simulink model "egnition_New_updated_shiva"  (R2019b)
settings: Solver=ode1  StartTime=0.0  StopTime=170  FixedStep=0.01  RelTol=1e-3
undefined symbols (not defined in the file or in its folder): BezierCurves, BezierLength, Constants, Driver, Ln, magnitude, v31
libraries: simulink_extras x3, simulink x2
(part 2 of 2)

== system egnition_New_updated_shiva/Tire Forces /Tire Model/co efficient of friction calculation ==
  "Resultant Slip " : Inport
  Fz : Inport  Port=2
  Bus Creator : BusCreator  Inputs=4
  Bus Creator1 : BusCreator  Inputs=4
  Bus Creator2 : BusCreator  Inputs=2
  Bus Selector : BusSelector  OutputSignals=Slip:L_FL,Slip:L_FR,Slip:L_RL,Slip:L_RR,Slip:S_FL,Slip:S_FR,Slip:S_RL,Slip:S_RR
  Bus Selector1 : BusSelector  OutputSignals=Resultant Slip FL,Resultant Slip FR,Resultant Slip RL,Resultant Slip RR
  Bus Selector2 : BusSelector  OutputSignals=Longitudinal_and_side_Slip,Resultant_Slip
  Bus Selector3 : BusSelector  OutputSignals=Fz_Dynamic.FZD_FL,Fz_Dynamic.FZD_FR,Fz_Dynamic.FZD_RL,Fz_Dynamic.FZD_RR
  Constant : Constant  Value=Constants.other_param.Friction_Tuning_Parameter
  Demux : Demux  Outputs=8
  MATLAB Code : MATLAB Function  TreatAsAtomicUnit=on
  Mew : Outport  VectorParamsAs1DForOutWhenUnconnected=off
  wires:
  Bus Selector2/1 -> Bus Selector/1  "<Longitudinal_and_side_Slip>"
  Bus Selector2/2 -> Bus Selector1/1  "<Resultant_Slip>"
  Bus Selector3/4 -> MATLAB Code/16(FZD_RR)  "<FZD_RR>"
  Bus Selector3/3 -> MATLAB Code/15(FZD_RL)  "<FZD_RL>"
  Bus Selector3/2 -> MATLAB Code/14(FZD_FR)  "<FZD_FR>"
  Bus Selector3/1 -> MATLAB Code/13(FZD_FL)  "<FZD_FL>"
  MATLAB Code/1(y) -> Demux/1
  Bus Selector1/1 -> MATLAB Code/9(SlipR_FL)  "<Resultant Slip FL>"
  Bus Selector1/2 -> MATLAB Code/10(SlipR_FR)  "<Resultant Slip FR>"
  Bus Selector1/3 -> MATLAB Code/11(SlipR_RL)  "<Resultant Slip RL>"
  Bus Selector1/4 -> MATLAB Code/12(SlipR_RR)  "<Resultant Slip RR>"
  Bus Selector/8 -> MATLAB Code/8(SlipS_RR)  "<Slip:S_RR>"
  Bus Selector/7 -> MATLAB Code/7(SlipS_RL)  "<Slip:S_RL>"
  Bus Selector/6 -> MATLAB Code/6(SlipS_FR)  "<Slip:S_FR>"
  Bus Selector/5 -> MATLAB Code/5(SlipS_FL)  "<Slip:S_FL>"
  Bus Selector/4 -> MATLAB Code/4(SlipL_RR)  "<Slip:L_RR>"
  Bus Selector/3 -> MATLAB Code/3(SlipL_RL)  "<Slip:L_RL>"
  Bus Selector/2 -> MATLAB Code/2(SlipL_FR)  "<Slip:L_FR>"
  Bus Selector/1 -> MATLAB Code/1(SlipL_FL)  "<Slip:L_FL>"
  Bus Creator/1 -> Bus Creator2/1  "Mew(l)"
  Bus Creator1/1 -> Bus Creator2/2  "Mew(s)"
  Bus Creator2/1 -> Mew/1
  "Resultant Slip "/1 -> Bus Selector2/1
  Demux/1 -> Bus Creator/1  "Mew(l)_FL"
  Demux/2 -> Bus Creator/2  "Mew(l)_FR"
  Demux/3 -> Bus Creator/3  "Mew(l)_RL"
  Demux/4 -> Bus Creator/4  "Mew(l)_RR"
  Demux/5 -> Bus Creator1/1  "Mew(s)_FL"
  Demux/6 -> Bus Creator1/2  "Mew(s)_FR"
  Demux/7 -> Bus Creator1/3  "Mew(s)_RL"
  Demux/8 -> Bus Creator1/4  "Mew(s)_RR"
  Constant/1 -> MATLAB Code/17(Friction_Tuning_parameter)
  Fz/1 -> Bus Selector3/1

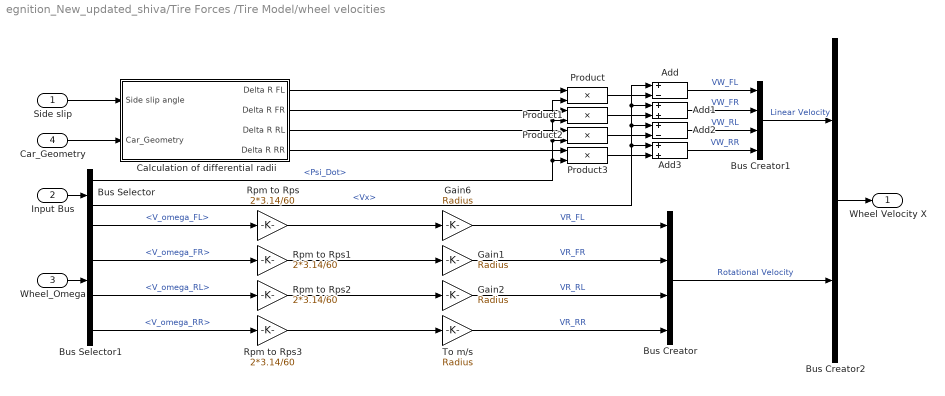
== system egnition_New_updated_shiva/Tire Forces /Tire Model/wheel velocities  ==
  "Side slip " : Inport
  Input Bus : Inport  Port=2
  Wheel_Omega : Inport  Port=3
  Car_Geometry : Inport  Port=4
  Add : Sum  Inputs=+-
  Add1 : Sum
  Add2 : Sum  Inputs=+-
  Add3 : Sum
  Bus Creator : BusCreator  Inputs=4
  Bus Creator1 : BusCreator  Inputs=4
  Bus Creator2 : BusCreator  Inputs=2
  Bus Selector : BusSelector  OutputSignals=Velocity.Psi_Dot,Velocity.Vx
  Bus Selector1 : BusSelector  OutputSignals=V_omega_FL,V_omega_FR,V_omega_RL,V_omega_RR
  Calculation of differential radii : Subsystem
  Gain1 : Gain  Gain=Radius
  Gain2 : Gain  Gain=Radius
  Gain6 : Gain  Gain=Radius
  Product{,1..3} (4 alike) : Product
  Rpm to Rps{,1..3} (4 alike) : Gain  Gain=2*3.14/60
  To m/s : Gain  Gain=Radius
  Wheel Velocity X : Outport  VectorParamsAs1DForOutWhenUnconnected=off
  wires:
  Car_Geometry/1 -> Calculation of differential radii/2(Car_Geometry)
  Wheel_Omega/1 -> Bus Selector1/1
  To m/s/1 -> Bus Creator/4  "VR_RR"
  Gain2/1 -> Bus Creator/3  "VR_RL"
  Gain1/1 -> Bus Creator/2  "VR_FR"
  Gain6/1 -> Bus Creator/1  "VR_FL"
  Input Bus/1 -> Bus Selector/1
  Add3/1 -> Bus Creator1/4  "VW_RR"
  Add2/1 -> Bus Creator1/3  "VW_RL"
  Add1/1 -> Bus Creator1/2  "VW_FR"
  Add/1 -> Bus Creator1/1  "VW_FL"
  Bus Selector/2 -> Add3/1, Add2/1, Add1/1, Add/1  "<Vx>"
  Product3/1 -> Add3/2
  Product2/1 -> Add2/2
  Product1/1 -> Add1/2
  Product/1 -> Add/2
  Bus Selector/1 -> Product3/2, Product2/2, Product1/2, Product/2  "<Psi_Dot>"
  Calculation of differential radii/4(Delta R RR) -> Product3/1
  Calculation of differential radii/3(Delta R RL) -> Product2/1
  Calculation of differential radii/2(Delta R FR) -> Product1/1
  Calculation of differential radii/1(Delta R FL) -> Product/1
  "Side slip "/1 -> Calculation of differential radii/1(Side slip angle)
  Bus Creator1/1 -> Bus Creator2/1  "Linear Velocity"
  Bus Creator/1 -> Bus Creator2/2  "Rotational Velocity"
  Bus Creator2/1 -> Wheel Velocity X/1
  Bus Selector1/1 -> Rpm to Rps/1  "<V_omega_FL>"
  Bus Selector1/2 -> Rpm to Rps1/1  "<V_omega_FR>"
  Bus Selector1/3 -> Rpm to Rps2/1  "<V_omega_RL>"
  Bus Selector1/4 -> Rpm to Rps3/1  "<V_omega_RR>"
  Rpm to Rps/1 -> Gain6/1
  Rpm to Rps1/1 -> Gain1/1
  Rpm to Rps2/1 -> Gain2/1
  Rpm to Rps3/1 -> To m/s/1

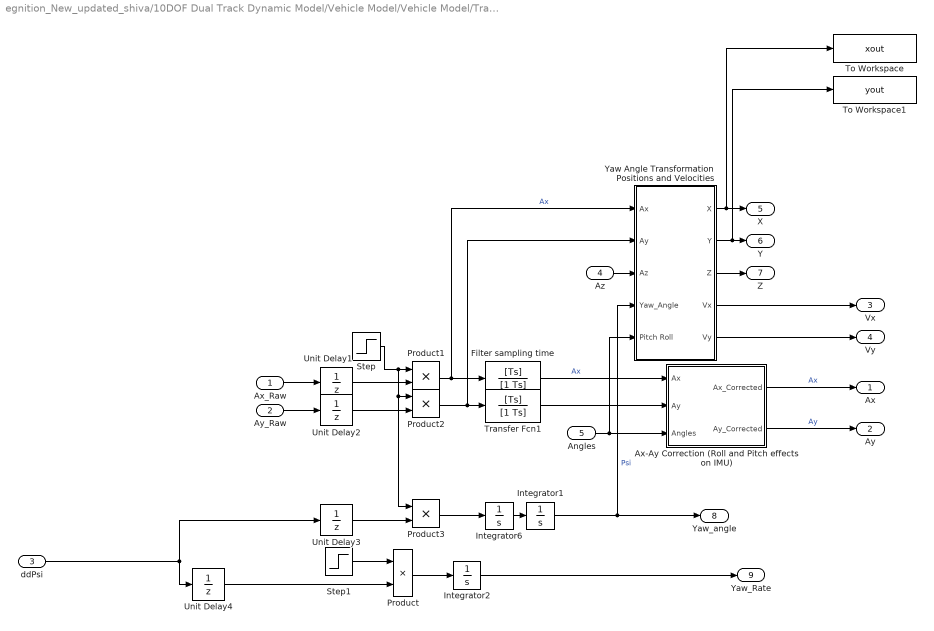
== system egnition_New_updated_shiva/10DOF Dual Track Dynamic Model/Vehicle Model/Vehicle Model/Transformation from Raw States to Car States ==
  Ax_Raw : Inport
  Ay_Raw : Inport  Port=2
  ddPsi : Inport  Port=3
  Az : Inport  Port=4
  Angles : Inport  Port=5
  Ax-Ay Correction (Roll and Pitch effects on IMU) : Subsystem
  Filter sampling time : TransferFcn  Numerator=[Ts]  Denominator=[1 Ts]
  Integrator1 : Integrator
  Integrator2 : Integrator  InitialCondition=0.0000000001
  Integrator6 : Integrator
  Product{,1..3} (4 alike) : Product
  Step : Step  Time=2
  Step1 : Step  Time=2.00000
  To Workspace : ToWorkspace  VariableName=xout  SampleTime=-1
  To Workspace1 : ToWorkspace  VariableName=yout  SampleTime=-1
  Transfer Fcn1 : TransferFcn  Numerator=[Ts]  Denominator=[1 Ts]
  Unit Delay1 : UnitDelay  SampleTime=-1  HasFrameUpgradeWarning=on
  Unit Delay2 : UnitDelay  SampleTime=-1  HasFrameUpgradeWarning=on
  Unit Delay3 : UnitDelay  SampleTime=-1  HasFrameUpgradeWarning=on
  Unit Delay4 : UnitDelay  InitialCondition=0.1  SampleTime=-1  HasFrameUpgradeWarning=on
  "Yaw Angle Transformation Positions and Velocities " : Subsystem
  Ax : Outport  VectorParamsAs1DForOutWhenUnconnected=off
  Ay : Outport  Port=2  VectorParamsAs1DForOutWhenUnconnected=off
  Vx : Outport  Port=3  VectorParamsAs1DForOutWhenUnconnected=off
  Vy : Outport  Port=4  VectorParamsAs1DForOutWhenUnconnected=off
  X : Outport  Port=5  VectorParamsAs1DForOutWhenUnconnected=off
  Y : Outport  Port=6  VectorParamsAs1DForOutWhenUnconnected=off
  Z : Outport  Port=7  VectorParamsAs1DForOutWhenUnconnected=off
  Yaw_angle : Outport  Port=8  VectorParamsAs1DForOutWhenUnconnected=off
  Yaw_Rate : Outport  Port=9  VectorParamsAs1DForOutWhenUnconnected=off
  wires:
  Ax-Ay Correction (Roll and Pitch effects on IMU)/2("Ay_Corrected ") -> Ay/1  "Ay"
  Ax-Ay Correction (Roll and Pitch effects on IMU)/1(Ax_Corrected) -> Ax/1  "Ax"
  Integrator2/1 -> Yaw_Rate/1
  Product/1 -> Integrator2/1
  Unit Delay4/1 -> Product/2
  ddPsi/1 -> Unit Delay3/1, Unit Delay4/1
  "Yaw Angle Transformation Positions and Velocities "/3(Z) -> Z/1
  Az/1 -> "Yaw Angle Transformation Positions and Velocities "/3("Az ")
  Unit Delay1/1 -> Product1/2
  Unit Delay2/1 -> Product2/2
  Unit Delay3/1 -> Product3/2
  Step/1 -> Product1/1, Product2/1, Product3/1
  Product3/1 -> Integrator6/1
  Ax_Raw/1 -> Unit Delay1/1
  Ay_Raw/1 -> Unit Delay2/1
  Integrator6/1 -> Integrator1/1
  "Yaw Angle Transformation Positions and Velocities "/2(Y) -> To Workspace1/1, Y/1
  "Yaw Angle Transformation Positions and Velocities "/1(X) -> To Workspace/1, X/1
  Integrator1/1 -> "Yaw Angle Transformation Positions and Velocities "/4(Yaw_Angle), Yaw_angle/1  "Psi"
  Step1/1 -> Product/1
  Product1/1 -> Filter sampling time/1, "Yaw Angle Transformation Positions and Velocities "/1(Ax)  "Ax"
  Angles/1 -> Ax-Ay Correction (Roll and Pitch effects on IMU)/3("Angles "), "Yaw Angle Transformation Positions and Velocities "/5("Pitch Roll ")
  Product2/1 -> Transfer Fcn1/1, "Yaw Angle Transformation Positions and Velocities "/2(Ay)
  Filter sampling time/1 -> Ax-Ay Correction (Roll and Pitch effects on IMU)/1(Ax)  "Ax"
  Transfer Fcn1/1 -> Ax-Ay Correction (Roll and Pitch effects on IMU)/2(Ay)
  "Yaw Angle Transformation Positions and Velocities "/4(Vx) -> Vx/1
  "Yaw Angle Transformation Positions and Velocities "/5(Vy) -> Vy/1

== system egnition_New_updated_shiva/Driver Model/lateral Controller/Subsystem/dynamic Stanely ==
  ey : Inport
  v : Inport  Port=2
  r_meas : Inport  Port=3
  r_trj : Inport  Port=4
  Yaw_c : Inport  Port=5
  Corrective_dynamic_Terms : Subsystem
  IC : InitialCondition  Value=0
  Kinematic_controller : Subsystem
  Radians to Degrees1 : simulink_extras/Transformations/Radians to Degrees
  Sum1 : Sum  Inputs=|++
  dynamic_steer : Outport
  wires:
  r_meas/1 -> Corrective_dynamic_Terms/1(r_meas)
  r_trj/1 -> Corrective_dynamic_Terms/5(r_trj)
  Corrective_dynamic_Terms/1(steer_correction) -> Sum1/2
  Sum1/1 -> Radians to Degrees1/1, Corrective_dynamic_Terms/2(steer)
  ey/1 -> Kinematic_controller/1(ey)
  v/1 -> Kinematic_controller/2(v), Corrective_dynamic_Terms/4(v)
  Kinematic_controller/1(delta_fb) -> Sum1/1
  Yaw_c/1 -> Corrective_dynamic_Terms/3(yaw_c)
  Radians to Degrees1/1 -> IC/1
  IC/1 -> dynamic_steer/1

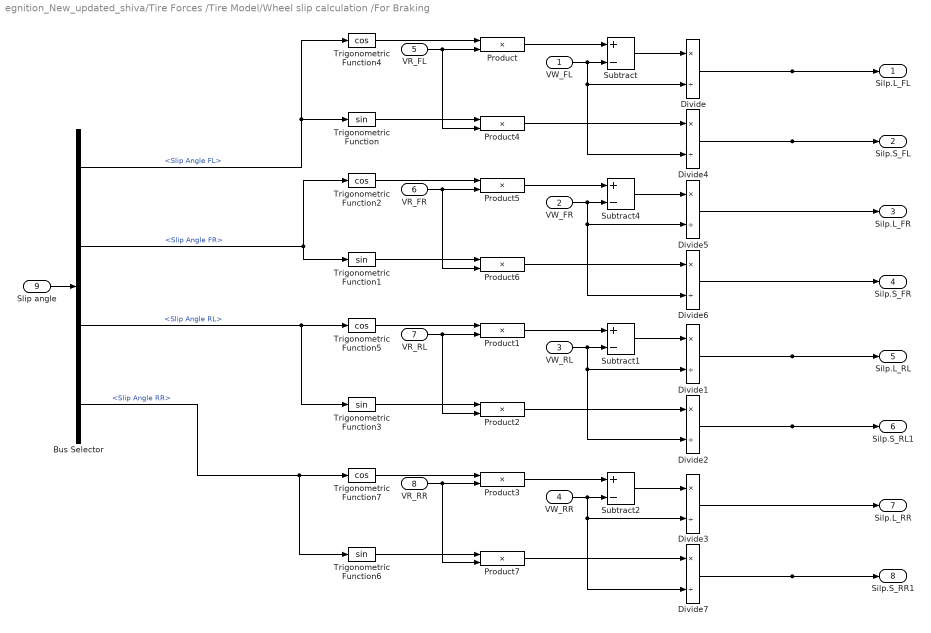
== system egnition_New_updated_shiva/Tire Forces /Tire Model/Wheel slip calculation /For Braking ==
  "VW_FL " : Inport
  VW_FR : Inport  Port=2
  VW_RL : Inport  Port=3
  VW_RR : Inport  Port=4
  VR_FL : Inport  Port=5
  VR_FR : Inport  Port=6
  VR_RL : Inport  Port=7
  "VR_RR " : Inport  Port=8
  "Slip angle " : Inport  Port=9
  Bus Selector : BusSelector  OutputSignals=Slip Angle FL,Slip Angle FR,Slip Angle RL,Slip Angle RR
  Divide{,1..7} (8 alike) : Product  Inputs=*/
  Product{,1..7} (8 alike) : Product
  Subtract{,1..2,4} (4 alike) : Sum  Inputs=+-
  Trigonometric Function{,1,3,6} (4 alike) : Trigonometry
  Trigonometric Function{2,4..5,7} (4 alike) : Trigonometry  Operator=cos
  Silp.L_FL : Outport  VectorParamsAs1DForOutWhenUnconnected=off
  Silp.S_FL : Outport  Port=2  VectorParamsAs1DForOutWhenUnconnected=off
  Silp.L_FR : Outport  Port=3  VectorParamsAs1DForOutWhenUnconnected=off
  Silp.S_FR : Outport  Port=4  VectorParamsAs1DForOutWhenUnconnected=off
  Silp.L_RL : Outport  Port=5  VectorParamsAs1DForOutWhenUnconnected=off
  Silp.S_RL1 : Outport  Port=6  VectorParamsAs1DForOutWhenUnconnected=off
  Silp.L_RR : Outport  Port=7  VectorParamsAs1DForOutWhenUnconnected=off
  Silp.S_RR1 : Outport  Port=8  VectorParamsAs1DForOutWhenUnconnected=off
  wires:
  "Slip angle "/1 -> Bus Selector/1
  Bus Selector/4 -> Trigonometric Function6/1, Trigonometric Function7/1  "<Slip Angle RR>"
  VW_RR/1 -> Subtract2/2, Divide3/2, Divide7/2
  Product7/1 -> Divide7/1
  "VR_RR "/1 -> Product3/2, Product7/2
  Product3/1 -> Subtract2/1
  Trigonometric Function6/1 -> Product7/1
  Subtract2/1 -> Divide3/1
  Trigonometric Function7/1 -> Product3/1
  VW_RL/1 -> Subtract1/2, Divide1/2, Divide2/2
  Product2/1 -> Divide2/1
  VR_RL/1 -> Product1/2, Product2/2
  Product1/1 -> Subtract1/1
  Trigonometric Function3/1 -> Product2/1
  Subtract1/1 -> Divide1/1
  Bus Selector/3 -> Trigonometric Function5/1, Trigonometric Function3/1  "<Slip Angle RL>"
  Trigonometric Function5/1 -> Product1/1
  Product5/1 -> Subtract4/1
  VW_FR/1 -> Subtract4/2, Divide5/2, Divide6/2
  Bus Selector/2 -> Trigonometric Function1/1, Trigonometric Function2/1  "<Slip Angle FR>"
  Trigonometric Function2/1 -> Product5/1
  VR_FR/1 -> Product5/2, Product6/2
  Subtract4/1 -> Divide5/1
  Trigonometric Function1/1 -> Product6/1
  Product6/1 -> Divide6/1
  Product4/1 -> Divide4/1
  Trigonometric Function/1 -> Product4/1
  "VW_FL "/1 -> Subtract/2, Divide/2, Divide4/2
  Product/1 -> Subtract/1
  Subtract/1 -> Divide/1
  VR_FL/1 -> Product/2, Product4/2
  Bus Selector/1 -> Trigonometric Function/1, Trigonometric Function4/1  "<Slip Angle FL>"
  Trigonometric Function4/1 -> Product/1
  Divide/1 -> Silp.L_FL/1
  Divide4/1 -> Silp.S_FL/1
  Divide5/1 -> Silp.L_FR/1
  Divide6/1 -> Silp.S_FR/1
  Divide1/1 -> Silp.L_RL/1
  Divide2/1 -> Silp.S_RL1/1
  Divide3/1 -> Silp.L_RR/1
  Divide7/1 -> Silp.S_RR1/1

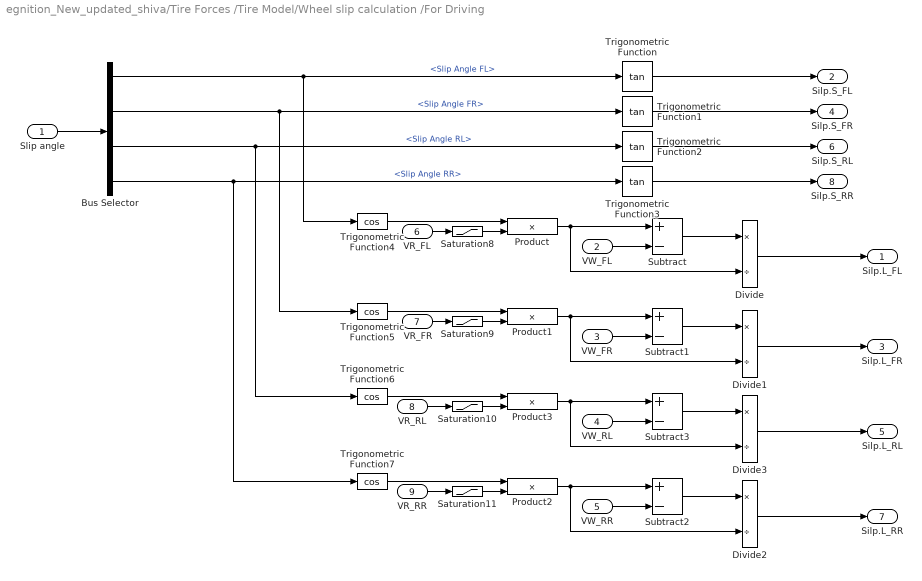
== system egnition_New_updated_shiva/Tire Forces /Tire Model/Wheel slip calculation /For Driving ==
  "Slip angle " : Inport
  "VW_FL " : Inport  Port=2
  VW_FR : Inport  Port=3
  VW_RL : Inport  Port=4
  VW_RR : Inport  Port=5
  VR_FL : Inport  Port=6
  VR_FR : Inport  Port=7
  VR_RL : Inport  Port=8
  "VR_RR " : Inport  Port=9
  Bus Selector : BusSelector  OutputSignals=Slip Angle FL,Slip Angle FR,Slip Angle RL,Slip Angle RR
  Divide{,1..3} (4 alike) : Product  Inputs=*/
  Product{,1..3} (4 alike) : Product
  Saturation{8..11} (4 alike) : Saturate  UpperLimit=500  LowerLimit=0.1
  Subtract{,1..3} (4 alike) : Sum  Inputs=+-
  Trigonometric Function{,1..3} (4 alike) : Trigonometry  Operator=tan
  Trigonometric Function{4..7} (4 alike) : Trigonometry  Operator=cos
  Silp.L_FL : Outport  VectorParamsAs1DForOutWhenUnconnected=off
  Silp.S_FL : Outport  Port=2  VectorParamsAs1DForOutWhenUnconnected=off
  Silp.L_FR : Outport  Port=3  VectorParamsAs1DForOutWhenUnconnected=off
  Silp.S_FR : Outport  Port=4  VectorParamsAs1DForOutWhenUnconnected=off
  Silp.L_RL : Outport  Port=5  VectorParamsAs1DForOutWhenUnconnected=off
  Silp.S_RL : Outport  Port=6  VectorParamsAs1DForOutWhenUnconnected=off
  Silp.L_RR : Outport  Port=7  VectorParamsAs1DForOutWhenUnconnected=off
  Silp.S_RR : Outport  Port=8  VectorParamsAs1DForOutWhenUnconnected=off
  wires:
  Saturation11/1 -> Product2/2
  Saturation10/1 -> Product3/2
  Saturation9/1 -> Product1/2
  Saturation8/1 -> Product/2
  Divide2/1 -> Silp.L_RR/1
  Divide3/1 -> Silp.L_RL/1
  Divide1/1 -> Silp.L_FR/1
  Divide/1 -> Silp.L_FL/1
  Trigonometric Function3/1 -> Silp.S_RR/1
  Trigonometric Function2/1 -> Silp.S_RL/1
  Trigonometric Function1/1 -> Silp.S_FR/1
  Trigonometric Function/1 -> Silp.S_FL/1
  "Slip angle "/1 -> Bus Selector/1
  Trigonometric Function5/1 -> Product1/1
  Product3/1 -> Subtract3/1, Divide3/2
  Trigonometric Function7/1 -> Product2/1
  VW_RR/1 -> Subtract2/2
  Product2/1 -> Subtract2/1, Divide2/2
  "VR_RR "/1 -> Saturation11/1
  Product1/1 -> Subtract1/1, Divide1/2
  Trigonometric Function6/1 -> Product3/1
  VR_RL/1 -> Saturation10/1
  Subtract1/1 -> Divide1/1
  Subtract2/1 -> Divide2/1
  VR_FR/1 -> Saturation9/1
  VW_RL/1 -> Subtract3/2
  VW_FR/1 -> Subtract1/2
  Subtract3/1 -> Divide3/1
  "VW_FL "/1 -> Subtract/2
  Product/1 -> Subtract/1, Divide/2
  Subtract/1 -> Divide/1
  VR_FL/1 -> Saturation8/1
  Bus Selector/4 -> Trigonometric Function3/1, Trigonometric Function7/1  "<Slip Angle RR>"
  Bus Selector/3 -> Trigonometric Function2/1, Trigonometric Function6/1  "<Slip Angle RL>"
  Bus Selector/2 -> Trigonometric Function1/1, Trigonometric Function5/1  "<Slip Angle FR>"
  Bus Selector/1 -> Trigonometric Function/1, Trigonometric Function4/1  "<Slip Angle FL>"
  Trigonometric Function4/1 -> Product/1

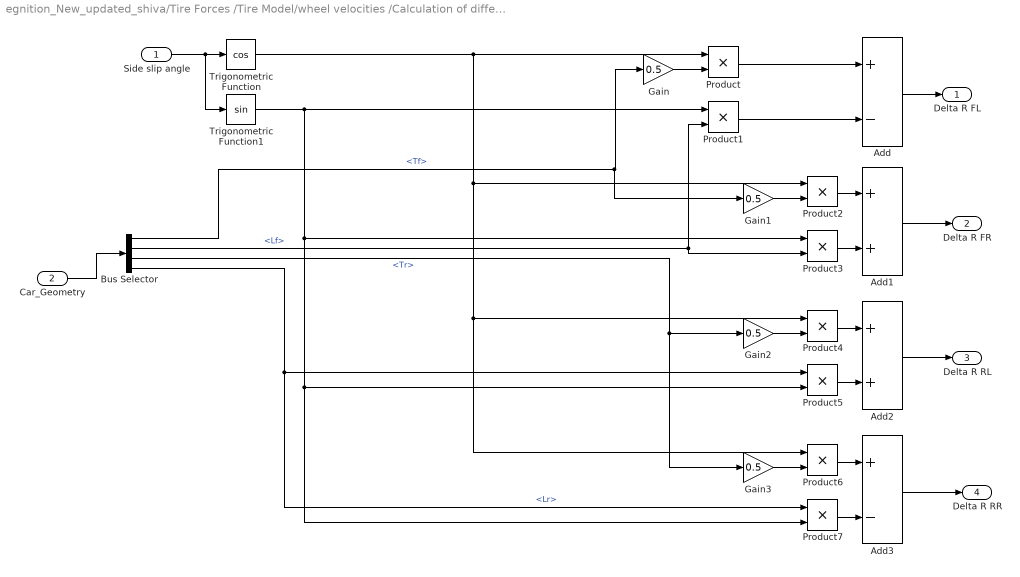
== system egnition_New_updated_shiva/Tire Forces /Tire Model/wheel velocities /Calculation of differential radii ==
  Side slip angle : Inport
  Car_Geometry : Inport  Port=2
  Add : Sum  Inputs=+-
  Add1 : Sum
  Add2 : Sum
  Add3 : Sum  Inputs=+-
  Bus Selector : BusSelector  OutputSignals=Tf,Lf,Tr,Lr
  Gain{,1..3} (4 alike) : Gain  Gain=0.5
  Product{,1..7} (8 alike) : Product
  Trigonometric Function : Trigonometry  Operator=cos
  Trigonometric Function1 : Trigonometry
  Delta R FL : Outport  VectorParamsAs1DForOutWhenUnconnected=off
  Delta R FR : Outport  Port=2  VectorParamsAs1DForOutWhenUnconnected=off
  Delta R RL : Outport  Port=3  VectorParamsAs1DForOutWhenUnconnected=off
  Delta R RR : Outport  Port=4  VectorParamsAs1DForOutWhenUnconnected=off
  wires:
  Car_Geometry/1 -> Bus Selector/1
  Add3/1 -> Delta R RR/1
  Add2/1 -> Delta R RL/1
  Add1/1 -> Delta R FR/1
  Add/1 -> Delta R FL/1
  Bus Selector/4 -> Product5/1, Product7/1  "<Lr>"
  Bus Selector/3 -> Gain2/1, Gain3/1  "<Tr>"
  Gain3/1 -> Product6/2
  Product6/1 -> Add3/1
  Product7/1 -> Add3/2
  Gain2/1 -> Product4/2
  Product4/1 -> Add2/1
  Product5/1 -> Add2/2
  Gain1/1 -> Product2/2
  Product2/1 -> Add1/1
  Product3/1 -> Add1/2
  Product/1 -> Add/1
  Product1/1 -> Add/2
  Trigonometric Function1/1 -> Product1/1, Product3/1, Product7/2, Product5/2
  Bus Selector/2 -> Product1/2, Product3/2  "<Lf>"
  Trigonometric Function/1 -> Product/1, Product2/1, Product6/1, Product4/1
  Gain/1 -> Product/2
  Bus Selector/1 -> Gain/1, Gain1/1  "<Tf>"
  Side slip angle/1 -> Trigonometric Function/1, Trigonometric Function1/1

== system egnition_New_updated_shiva/10DOF Dual Track Dynamic Model/Vehicle Model/Vehicle Model/Transformation from Raw States to Car States/Ax-Ay Correction (Roll and Pitch effects on IMU) ==
  Ax : Inport
  Ay : Inport  Port=2
  "Angles " : Inport  Port=3
  Add : Sum
  Add1 : Sum  Inputs=+-
  Bus Selector : BusSelector  OutputSignals=Theta,Phi
  Cos : Trigonometry  Operator=cos
  Gain : Gain  Gain=9.81
  Gain1 : Gain  Gain=9.81
  Product : Product
  Sin : Trigonometry
  Sin1 : Trigonometry
  Ax_Corrected : Outport  VectorParamsAs1DForOutWhenUnconnected=off
  "Ay_Corrected " : Outport  Port=2  VectorParamsAs1DForOutWhenUnconnected=off
  wires:
  "Angles "/1 -> Bus Selector/1
  Bus Selector/1 -> Sin/1, Cos/1  "<Theta>"
  Bus Selector/2 -> Sin1/1  "<Phi>"
  Ax/1 -> Add/1
  Sin/1 -> Gain/1
  Gain/1 -> Add/2
  Cos/1 -> Product/1
  Sin1/1 -> Product/2
  Gain1/1 -> Add1/2
  Ay/1 -> Add1/1
  Add/1 -> Ax_Corrected/1
  Add1/1 -> "Ay_Corrected "/1
  Product/1 -> Gain1/1

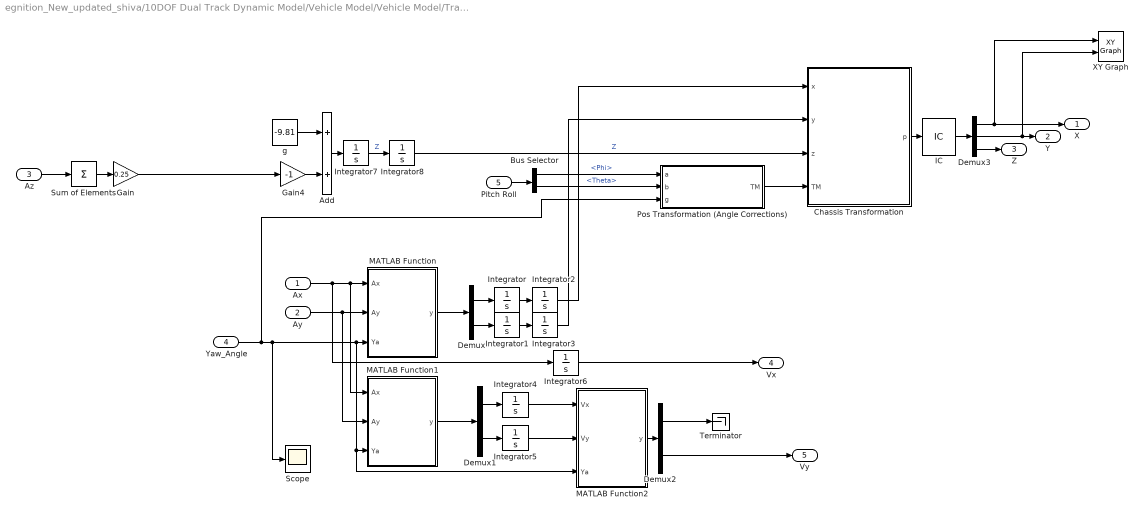
== system egnition_New_updated_shiva/10DOF Dual Track Dynamic Model/Vehicle Model/Vehicle Model/Transformation from Raw States to Car States/Yaw Angle Transformation Positions and Velocities  ==
  Ax : Inport
  Ay : Inport  Port=2
  "Az " : Inport  Port=3
  Yaw_Angle : Inport  Port=4
  "Pitch Roll " : Inport  Port=5
  Add : Sum
  Bus Selector : BusSelector  OutputSignals=Phi,Theta
  Chassis Transformation : MATLAB Function  TreatAsAtomicUnit=on
  Demux : Demux  Outputs=2
  Demux1 : Demux  Outputs=2
  Demux2 : Demux  Outputs=2
  Demux3 : Demux  Outputs=3
  Gain : Gain  Gain=0.25
  Gain4 : Gain  Gain=-1
  IC : InitialCondition  Value=[Constants.initial_param.X0;Constants.initial_param.Y0;Constants.initial_param.Z0]
  Integrator{,1,4..5,7} (5 alike) : Integrator
  Integrator2 : Integrator  InitialCondition=Constants.initial_param.X0
  Integrator3 : Integrator  InitialCondition=Constants.initial_param.Y0
  Integrator6 : Integrator  InitialCondition=0.1
  Integrator8 : Integrator  InitialCondition=Constants.initial_param.Z0
  MATLAB Function : MATLAB Function  TreatAsAtomicUnit=on
  MATLAB Function1 : MATLAB Function  TreatAsAtomicUnit=on
  MATLAB Function2 : MATLAB Function  TreatAsAtomicUnit=on
  "Pos Transformation (Angle Corrections) " : MATLAB Function  TreatAsAtomicUnit=on
  Scope : Scope
  Sum of Elements : Sum  Inputs=+
  Terminator : Terminator
  XY Graph : simulink/Sinks/XY Graph  xmin=xy.Xmin  xmax=xy.Xmax  ymin=xy.Ymin  ymax=xy.Ymax  st=0.1
  g : Constant  Value=-9.81
  X : Outport  VectorParamsAs1DForOutWhenUnconnected=off
  Y : Outport  Port=2  VectorParamsAs1DForOutWhenUnconnected=off
  Z : Outport  Port=3  VectorParamsAs1DForOutWhenUnconnected=off
  Vx : Outport  Port=4  VectorParamsAs1DForOutWhenUnconnected=off
  Vy : Outport  Port=5  VectorParamsAs1DForOutWhenUnconnected=off
  wires:
  Gain/1 -> Gain4/1
  Sum of Elements/1 -> Gain/1
  Demux2/2 -> Vy/1
  Integrator6/1 -> Vx/1
  Demux2/1 -> Terminator/1
  Demux3/2 -> XY Graph/2, Y/1
  Demux3/1 -> XY Graph/1, X/1
  "Pitch Roll "/1 -> Bus Selector/1
  "Az "/1 -> Sum of Elements/1
  Gain4/1 -> Add/2
  Integrator7/1 -> Integrator8/1  "Z"
  Add/1 -> Integrator7/1
  Integrator8/1 -> Chassis Transformation/3(z)  "Z"
  g/1 -> Add/1
  Demux3/3 -> Z/1
  Chassis Transformation/1(p) -> IC/1
  Integrator2/1 -> Chassis Transformation/1(x)
  Yaw_Angle/1 -> Scope/1, MATLAB Function1/3(Ya), MATLAB Function2/3(Ya), MATLAB Function/3(Ya), "Pos Transformation (Angle Corrections) "/3(g)
  Integrator3/1 -> Chassis Transformation/2(y)
  "Pos Transformation (Angle Corrections) "/1(TM) -> Chassis Transformation/4(TM)
  Bus Selector/1 -> "Pos Transformation (Angle Corrections) "/1(a)  "<Phi>"
  Bus Selector/2 -> "Pos Transformation (Angle Corrections) "/2(b)  "<Theta>"
  IC/1 -> Demux3/1
  Ax/1 -> Integrator6/1, MATLAB Function/1(Ax), MATLAB Function1/1(Ax)
  Ay/1 -> MATLAB Function/2(Ay), MATLAB Function1/2(Ay)
  MATLAB Function/1(y) -> Demux/1
  Demux/1 -> Integrator/1
  Demux/2 -> Integrator1/1
  Integrator1/1 -> Integrator3/1
  Integrator/1 -> Integrator2/1
  MATLAB Function2/1(y) -> Demux2/1
  Integrator4/1 -> MATLAB Function2/1(Vx)
  Integrator5/1 -> MATLAB Function2/2(Vy)
  Demux1/2 -> Integrator5/1
  Demux1/1 -> Integrator4/1
  MATLAB Function1/1(y) -> Demux1/1

== system egnition_New_updated_shiva/Driver Model/lateral Controller/Subsystem/dynamic Stanely/Corrective_dynamic_Terms ==
  r_meas : Inport
  steer : Inport  Port=2
  yaw_c : Inport  Port=3
  v : Inport  Port=4
  r_trj : Inport  Port=5
  Constant : Constant
  Gain : Gain  Gain=0
  Gain1 : Gain  Gain=0
  Gain2 : Gain
  Scope : Scope
  Stabilize_steer_delay : Subsystem
  Stabilize_yaw_dynamics : Subsystem
  Sum : Sum  Inputs=+++
  steadystate_yaw : Subsystem
  steer_correction : Outport
  wires:
  r_trj/1 -> steadystate_yaw/3(r_trj), Stabilize_yaw_dynamics/1(r_trj)
  v/1 -> steadystate_yaw/2(v)
  yaw_c/1 -> steadystate_yaw/1(yaw_c)
  r_meas/1 -> Stabilize_yaw_dynamics/2(r_meas)
  steer/1 -> Stabilize_steer_delay/1(steer_out)
  Sum/1 -> Scope/1, steer_correction/1
  steadystate_yaw/1(d1) -> Gain/1
  Stabilize_yaw_dynamics/1(d2) -> Gain1/1
  Constant/1 -> steadystate_yaw/Enable
  Stabilize_steer_delay/1(d3) -> Gain2/1
  Gain/1 -> Sum/1
  Gain1/1 -> Sum/2
  Gain2/1 -> Sum/3

== system egnition_New_updated_shiva/Driver Model/lateral Controller/Subsystem/dynamic Stanely/Kinematic_controller ==
  ey : Inport
  v : Inport  Port=2
  Product : Product  Inputs=**
  Scope : Scope
  Stanley Gain : Constant  Value=Constants.cont_param.k_stan
  Sum1 : Sum  Inputs=|++
  Trigonometric Function : Trigonometry  Operator=atan2
  soft_gain : Constant  Value=Constants.cont_param.k_soft
  delta_fb : Outport  VectorParamsAs1DForOutWhenUnconnected=off
  wires:
  v/1 -> Sum1/1
  Stanley Gain/1 -> Product/2
  ey/1 -> Product/1
  Trigonometric Function/1 -> Scope/1, delta_fb/1
  Sum1/1 -> Trigonometric Function/2
  soft_gain/1 -> Sum1/2
  Product/1 -> Trigonometric Function/1

== system egnition_New_updated_shiva/Driver Model/lateral Controller/Subsystem/dynamic Stanely/Corrective_dynamic_Terms/Stabilize_steer_delay ==
  steer_out : Inport
  Delay : Delay  InitialCondition=0.001
  Gain : Gain  Gain=Constants.cont_param.kd_steer*-1
  Sum : Sum  Inputs=|+-
  d3 : Outport
  wires:
  steer_out/1 -> Delay/1, Sum/2
  Delay/1 -> Sum/1
  Sum/1 -> Gain/1
  Gain/1 -> d3/1

== system egnition_New_updated_shiva/Driver Model/lateral Controller/Subsystem/dynamic Stanely/Corrective_dynamic_Terms/Stabilize_yaw_dynamics ==
  r_trj : Inport
  r_meas : Inport  Port=2
  Gain : Gain  Gain=Constants.cont_param.kd_yaw
  Sum : Sum  Inputs=-+
  d2 : Outport
  wires:
  r_trj/1 -> Sum/1
  r_meas/1 -> Sum/2
  Sum/1 -> Gain/1
  Gain/1 -> d2/1

== system egnition_New_updated_shiva/Driver Model/lateral Controller/Subsystem/dynamic Stanely/Corrective_dynamic_Terms/steadystate_yaw ==
  yaw_c : Inport
  v : Inport  Port=2
  r_trj : Inport  Port=3
  Enable : EnablePort
  Constant : Constant  Value=Constants.cont_param.k_ag/-1
  Divide : Product  Inputs=***
  Sum : Sum  Inputs=+-
  d1 : Outport
  wires:
  v/1 -> Divide/1
  r_trj/1 -> Divide/2
  Constant/1 -> Divide/3
  Divide/1 -> Sum/2  "yaw_ss"
  yaw_c/1 -> Sum/1
  Sum/1 -> d1/1

== matlab function egnition_New_updated_shiva/Engine_Model/MATLAB Function ==
  data: TP input; Requested_Torque output; BP input; T_peak input
function Requested_Torque = fcn(TP,BP,T_peak)
if BP==0
T=TP*T_peak;
else
T=-BP*T_peak;
end

Requested_Torque=T;

== matlab function egnition_New_updated_shiva/10DOF Dual Track Dynamic Model/Vehicle Model/Vehicle Model/Transformation from Raw States to Car States/Yaw Angle Transformation Positions and Velocities /Chassis Transformation ==
  data: x input; p output; y input; z input; TM input
function p  = fcn(x,y,z,TM)

p =[x-3.06;y;z]+TM*[3.06;0;0];

== matlab function egnition_New_updated_shiva/10DOF Dual Track Dynamic Model/Vehicle Model/Vehicle Model/Transformation from Raw States to Car States/Yaw Angle Transformation Positions and Velocities /Pos Transformation (Angle Corrections)  ==
  data: a input; TM output; b input; g input
function TM = Tranformation_Matrix(a,b,g)
TM_a = [1       0         0; 
            0 cos(a) -sin(a); 
            0 sin(a) cos(a)];
        
TM_b = [cos(b)     0   sin(b); 
                0         1       0    ; 
           -sin(b)     0   cos(b)];
       
TM_g = [cos(g) -sin(g)  0; 
            sin(g) cos(g)   0;
                0         0       1];
TM =TM_g*TM_b*TM_a;

== matlab function egnition_New_updated_shiva/Driver Model/lateral Controller/BezierPathReference ==
  data: ey output; eYaw output double; pCar input; yawCar input; tol input double; bezierCurves input; bezierLength input; kappa output; lengh output
function [ey,eYaw,kappa,lengh]  = doFrameConversion(pCar,yawCar,tol,bezierCurves,bezierLength)
    epsilon = 0.000000000000001;
    pTarget = [pCar(1),pCar(2),yawCar];
    numberOfCurves = numel(bezierCurves(1,1,:));
    distCurve = 1000 * ones(numberOfCurves,1);
    tCurve = zeros(numberOfCurves,1);
%     for i = previouseSpline-2:1:previouseSpline+2
    for i = 1:numberOfCurves
        curve = bezierCurves(:,:,mod(i-1,numberOfCurves)+1);
        %plotBezierCurves(curve, i -1);
        [tCurve(mod(i-1,numberOfCurves)+1),distCurve(mod(i-1,numberOfCurves)+1)] = findClosestPoint(curve,tol,pTarget(1:2));
    end
    [~,closedCurve] = min(distCurve);
    previouseSpline = 1;
    lengh = 0;
    step = 0.001;
    for i = 1:1:closedCurve - 1
        lengh = lengh + bezierLength(i);
    end
    lengh = lengh + calcLengthOfSegment(bezierCurves(:,:,closedCurve),step,tCurve(closedCurve));

    ey = distCurve(closedCurve);

    [kappa,dir] = calcKappaTangent(bezierCurves(:,:,closedCurve),tCurve(closedCurve));
    normalVec = [-dir(2),dir(1)];
    closestPoint = pointInCurve(bezierCurves(:,:,closedCurve),tCurve(closedCurve));
    if (norm(pTarget(1:2) - closestPoint)) < norm(pTarget(1:2) - closestPoint - epsilon * normalVec)
       ey = -ey; 
    end
    
    eYaw = pTarget(3) - atan2(dir(2),dir(1));
    while eYaw > pi
        eYaw = eYaw - 2 * pi;
    end
    while eYaw < -pi
        eYaw = eYaw + 2 * pi;
    end
%     eYaw = -eYaw;
    %% Calculate Kappa for next curves
    
    initDist = lengh;
    actDist = 0;
    i = closedCurve;

%     tstart = tCurve(closedCurve);
%     index = 1;
%     if distIteration < 10
%         distIteration = 10;
%     end
%     while actDist < distIteration
%         kappaS(index) = calcKappaTangent(bezierCurves(:,:,1 + mod(i - 1,numberOfCurves)),tstart);
%         distCov(index) = lengthTillCurve + calcLengthOfSegment(bezierCurves(:,:,1 + mod(i - 1,numberOfCurves)),step,tstart);
%         tstart = tstart + 0.0002 * index;
%         actDist = distCov(index) - initDist;
%         if tstart > 1
%             lengthTillCurve = lengthTillCurve + calcLengthOfSegment(bezierCurves(:,:,1 + mod(i - 1,numberOfCurves)),step,1);
%             tstart = tstart - 1;
%             i = i+1;
%         end
%         index = index + 1;
%     end
%     
%     distCov = distCov - distCov(1);
%     
% %     figure(1)
% %     hold on
% %     plot(distCov,kappaS);
%     kappaPol = polyfit(distCov,kappaS,5);
%     kappaSapprox = polyval(kappaPol,distCov);
%     plot(distCov,kappaSapprox)
end

%% DONT CHANGE ANYTHING DOWN HERE, JUST CHANGE THE FIRST PART IF NECCESARY


function [t,dist] = findClosestPoint(curve,tol,refPoint)
    t = 0.5;
    initPoint = pointInCurve(curve,t);
    dist = norm(initPoint - refPoint);
    h = 0.25;
    while h > tol
         tR = t + h;
         pR = pointInCurve(curve,tR);
         distR = norm(pR - refPoint);
         tL = t - h; 
         pL = pointInCurve(curve,tL);
         distL = norm(pL - refPoint);
         if distR < dist
             dist = distR;
             t = tR;
         elseif distL < dist
             dist = distL;
             t = tL;
         end
         h = h/2;
    end
end

function point = pointInCurve(curve,t)
    VecT = [1,t,t^2,t^3];
    Mat = [ 1  0  0  0;...
           -3  3  0  0;...
            3 -6  3  0;...
           -1  3 -3  1];
    point = VecT * Mat * curve;
end


function l = calcLengthOfSegment(curve,step,t)
%     subsec = 0:step:t;
%     pointsFirstDev = 3 * [curve(2,:) - curve(1,:); curve(3,:) - curve(2,:);curve(4,:) - curve(3,:)];
%     matT = ones(numel(subsec),4);
%     matT(:,2) = subsec';
%     matT(:,3) = subsec'.^2;
%     matT(:,4) = subsec'.^3;
%     convMat = [ 1  0  0  0;...
%                -3  3  0  0;...
%                 3 -6  3  0;...
%                -1  3 -3  1];
%     point = matT * convMat * curve;
%     l = 0;
%     for i = 1:numel(subsec)-1
%        l = l + norm(point(i,:) - point(i+1,:));
%     end
    
    subsec = 0:step:t;
    pointsFirstDev = 3 * [curve(2,:) - curve(1,:); curve(3,:) - curve(2,:);curve(4,:) - curve(3,:)];
    matT = ones(numel(subsec),3);
    matT(:,2) = subsec';
    matT(:,3) = subsec'.^2;
    convMat = [ 1  0  0;...
               -2  2  0;...
                1 -2  1];
    point = matT * convMat * pointsFirstDev;
    l = sum(sqrt(point(:,1).^2 + point(:,2).^2)) * step;
    
    %this function needs to be done in a more beautiful way.
end

function [kappa,dir] = calcKappaTangent(curve,t)
    if t == 0
        t = 0.0001;
    end
    if t == 1
        t = 0.9999;
    end
    pointsFirstDev = 3 * [curve(2,:) - curve(1,:); curve(3,:) - curve(2,:);curve(4,:) - curve(3,:)];
    matT = [1,t,t^2];
    convMat = [ 1  0  0;...
               -2  2  0;...
                1 -2  1];
    dev1 = matT * convMat * pointsFirstDev;
   
    pointsSecondDev = 2 * [pointsFirstDev(2,:) - pointsFirstDev(1,:); pointsFirstDev(3,:) - pointsFirstDev(2,:)];
    matT = [1,t];
    convMat = [ 1  0;...
                -1  1];
    dev2 = matT * convMat * pointsSecondDev;
    
    kappa = (dev1(1).*dev2(2) - dev1(2).*dev2(1)) ./ (dev1(1).^2 + dev1(2).^2).^(3/2);
    dir = dev1/norm(dev1);    
end

== matlab function egnition_New_updated_shiva/Normal Forces/Lx_Ly_Calculator/MATLAB Function ==
  data: W_FL input; y output; W_FR input; W_RL input; W_RR input; Wheel_Base input; Front_track input; Rear_track input
function y = fcn(W_FL,W_FR,W_RL,W_RR,Wheel_Base,Front_track,Rear_track)
Lx_FL=((W_RL*Wheel_Base)/(W_FL+W_RL));
Lx_FR=((W_RR*Wheel_Base)/(W_FR+W_RR));
Lx_RL=((W_FL*Wheel_Base)/(W_FL+W_RL));
Lx_RR=((W_FR*Wheel_Base)/(W_FR+W_RR));
Ly_FL=((W_FR*Front_track)/(W_FL+W_FR));
Ly_FR=((W_FL*Front_track)/(W_FL+W_FR));
Ly_RL=((W_RR*Rear_track)/(W_RL+W_RR));
Ly_RR=((W_RL*Rear_track)/(W_RL+W_RR));
y = [Lx_FL
     Lx_FR
     Lx_RL
     Lx_RR
     Ly_FL
     Ly_FR
     Ly_RL
     Ly_RR];

== matlab function egnition_New_updated_shiva/Tire Forces /Tire Model/Wheel Model1/Rolling Resistance ==
  data: Fr output; VW_FL input; VW_FR input; VW_RL input; VW_RR input; VR_FL input; VR_FR input; VR_RL input; VR_RR input; Fz_FL input; Fz_FR input; Fz_RL input; Fz_RR input; Radius input
function Fr = fcn(VW_FL,VW_FR,VW_RL,VW_RR,VR_FL,VR_FR,VR_RL,VR_RR,Fz_FL,Fz_FR,Fz_RL,Fz_RR,Radius)
c=0.03;
Fr_FL=c*(VW_FL*(0.980/2)/VR_FL)+(0.05+(0.01+0.0095*(VW_FL/100)*(VW_FL/100)))*Fz_FL*Radius;
Fr_FR=c*(VW_FR*(0.980/2)/VR_FR)+(0.05+(0.01+0.0095*(VW_FR/100)*(VW_FR/100)))*Fz_FR*Radius;
Fr_RL=c*(VW_RL*(0.980/2)/VR_RL)+(0.05+(0.01+0.0095*(VW_RL/100)*(VW_RL/100)))*Fz_RL*Radius;
Fr_RR=c*(VW_RR*(0.980/2)/VR_RR)+(0.05+(0.01+0.0095*(VW_RR/100)*(VW_RR/100)))*Fz_RR*Radius;

Fr=[Fr_FL
    Fr_FR
    Fr_RL
    Fr_RR];



% 
% c*(VW_FL*(0.980/2)/VR_FL)
% c*(VW_FR*(0.980/2)/VR_FR)
% c*(VW_RL*(0.980/2)/VR_RL)
% c*(VW_RR*(0.980/2)/VR_RR)

== matlab function egnition_New_updated_shiva/10DOF Dual Track Dynamic Model/Vehicle Model/Vehicle Model/Dual Track Equation of Motion ==
  data: Fx_FL input; y output; Fx_FR input; Fx_RL input; Fx_RR input; Fy_FL input; Fy_FR input; Fy_RL input; Fy_RR input; Mass input; Lf input; Lr input; Tf input; Tr input; Jz input; Delta input
function y = fcn(Fx_FL,Fx_FR,Fx_RL,Fx_RR,Fy_FL,Fy_FR,Fy_RL,Fy_RR,Mass,Lf,Lr,Tf,Tr,Jz,Delta)
Ax=(Fx_FL+Fx_FR)*cos(Delta)+Fx_RL+Fx_RR-(Fy_FL+Fy_FR)*sin(Delta);
Ay=(Fx_FL+Fx_FR)*sin(Delta)+(Fy_RL+Fy_RR)+(Fy_FL+Fy_FR)*cos(Delta);
Ya_A=(Tf/2)*(Fy_FL-Fy_FR)*sin(Delta)+Lf*(Fy_FL+Fy_FR)*cos(Delta)-Lr*(Fy_RL+Fy_RR)-(Tf/2)*(Fx_FL-Fx_FR)*cos(Delta)-Lf*(Fx_FL+Fx_FR)*sin(Delta)-(Tr/2)*(Fx_RL-Fx_RR);

y = [Ax/Mass
     Ay/Mass
     Ya_A/Jz];

== matlab function egnition_New_updated_shiva/10DOF Dual Track Dynamic Model/Vehicle Model/Vehicle Model/Transformation from Raw States to Car States/Yaw Angle Transformation Positions and Velocities /MATLAB Function ==
  data: Ax input; y output; Ay input; Ya input
function y = fcn(Ax,Ay,Ya)
Vx=Ax*cos(Ya)-Ay*sin(Ya);
Vy=Ax*sin(Ya)+Ay*cos(Ya);
y = [Vx
    Vy];

== matlab function egnition_New_updated_shiva/10DOF Dual Track Dynamic Model/Vehicle Model/Vehicle Model/Transformation from Raw States to Car States/Yaw Angle Transformation Positions and Velocities /MATLAB Function1 ==
  data: Ax input; y output; Ay input; Ya input
function y = fcn(Ax,Ay,Ya)
Vx=Ax*cos(Ya)-Ay*sin(Ya);
Vy=Ax*sin(Ya)+Ay*cos(Ya);
y = [Vx
    Vy];

== matlab function egnition_New_updated_shiva/10DOF Dual Track Dynamic Model/Vehicle Model/Vehicle Model/Transformation from Raw States to Car States/Yaw Angle Transformation Positions and Velocities /MATLAB Function2 ==
  data: Vx input; y output; Vy input; Ya input
function y = fcn(Vx,Vy,Ya)
Xdot=Vx*cos(Ya)+Vy*sin(Ya);
Ydot=-Vx*sin(Ya)+Vy*cos(Ya);
y = [Xdot
    Ydot];

== matlab function egnition_New_updated_shiva/Normal Forces/Longitudinal Dynamic Fz/MATLAB Function ==
  data: V_COG input; y output; Accel_X input; W input; C input; B input; H_COG input; Wb input
function y = fcn(V_COG,Accel_X,W,C,B,H_COG,Wb)
Wf=(W*C*9.81-W*H_COG*Accel_X)/Wb+(0.9288*V_COG*V_COG);
Wr=(W*B*9.81+W*H_COG*Accel_X)/Wb+(0.828*V_COG*V_COG);
WFL=Wf/2;
WRR=Wr/2;

y =[WFL
    WRR];
end

== matlab function egnition_New_updated_shiva/Normal Forces/Lateral Dynamic Fz/MATLAB Function ==
  data: Sprung_Mass input; y output; distance_sprung_mass_cg_and_roll_axis input; front_roll_stiffness input; rear_roll_stiffness input; mass_of_car input; Accel_Y input
function y = fcn(Sprung_Mass,distance_sprung_mass_cg_and_roll_axis,front_roll_stiffness,rear_roll_stiffness,mass_of_car,Accel_Y)
Roll_Angle=(Sprung_Mass*distance_sprung_mass_cg_and_roll_axis*Accel_Y)/(front_roll_stiffness+rear_roll_stiffness-(mass_of_car*distance_sprung_mass_cg_and_roll_axis));
y = Roll_Angle;

== matlab function egnition_New_updated_shiva/Tire Forces /Tire Model/Lateral Forces/MATLAB Function ==
  data: SA_FL input; y output; SA_FR input; SA_RL input; SA_RR input; MewL_FL input; MewL_FR input; MewL_RL input; MewL_RR input; MewS_FL input; MewS_FR input; MewS_RL input; MewS_RR input; FZ_FL input; FZ_FR input; FZ_RL input; FZ_RR input; Steering_Angle input
function y = fcn(SA_FL,SA_FR,SA_RL,SA_RR,MewL_FL,MewL_FR,MewL_RL,MewL_RR,MewS_FL,MewS_FR,MewS_RL,MewS_RR,FZ_FL,FZ_FR,FZ_RL,FZ_RR,Steering_Angle)
%% Frictional Force In global co ordinate system
% Longitudinal Directional Frictional forces 
Fwl_FL=MewL_FL*FZ_FL;
Fwl_FR=MewL_FR*FZ_FR;
Fwl_RL=MewL_RL*FZ_RL;
Fwl_RR=MewL_RR*FZ_RR;
% Lateral Directional Frictional forces 
Fws_FL=MewS_FL*FZ_FL;
Fws_FR=MewS_FR*FZ_FR;
Fws_RL=MewS_RL*FZ_RL;
Fws_RR=MewS_RR*FZ_RR;
%% transformed into the wheel coordinate system:
% Longitudinal Directional Frictional forces
Fl_FL=Fwl_FL*cos(SA_FL)+Fws_FL*sin(SA_FL);
Fl_FR=Fwl_FR*cos(SA_FR)+Fws_FR*sin(SA_FR);
Fl_RL=Fwl_RL*cos(SA_RL)+Fws_RL*sin(SA_RL);
Fl_RR=Fwl_RR*cos(SA_RR)+Fws_RR*sin(SA_RR);
% Lateral Directional Frictional forces 
Fs_FL=Fws_FL*cos(SA_FL)-Fwl_FL*sin(SA_FL);
Fs_FR=Fws_FR*cos(SA_FR)-Fwl_FR*sin(SA_FR);
Fs_RL=Fws_RL*cos(SA_RL)-Fwl_RL*sin(SA_RL);
Fs_RR=Fws_RR*cos(SA_RR)-Fwl_RR*sin(SA_RR);
%% translation all four steering angleare considered:
Fy_FL=Fs_FL*cos(Steering_Angle)+Fl_FL*sin(Steering_Angle);
Fy_FR=Fs_FR*cos(Steering_Angle)+Fl_FR*sin(Steering_Angle);
Fy_RL=Fs_RL;
Fy_RR=Fs_RR;

y =[Fy_FL
    Fy_FR
    Fy_RL
    Fy_RR
    Fws_FL
    Fws_FR
    Fws_RL
    Fws_RR
    Fwl_FL
    Fwl_FR
    Fwl_RL
    Fwl_RR];

== matlab function egnition_New_updated_shiva/Tire Forces /Tire Model/ Longitudinal  Force/MATLAB Function ==
  data: Steering_Angle input; y output; Fws_FL input; Fws_FR input; Fws_RL input; Fws_RR input; Fwl_FL input; Fwl_FR input; Fwl_RL input; Fwl_RR input; SA_FL input; SA_FR input; SA_RL input; SA_RR input
function y = fcn(Steering_Angle,Fws_FL,Fws_FR,Fws_RL,Fws_RR,Fwl_FL,Fwl_FR,Fwl_RL,Fwl_RR,SA_FL,SA_FR,SA_RL,SA_RR)
%%  transformed into the wheel coordinate system
Fl_FL= Fwl_FL*cos(SA_FL)+Fws_FL*sin(SA_FL);
Fl_FR= Fwl_FR*cos(SA_FR)+Fws_FR*sin(SA_FR);
Fl_RL= Fwl_RL*cos(SA_RL)+Fws_RL*sin(SA_RL);
Fl_RR= Fwl_RR*cos(SA_RR)+Fws_RR*sin(SA_RR);

Fs_FL= Fws_FL*cos(SA_FL)-Fwl_FL*sin(SA_FL);
Fs_FR= Fws_FR*cos(SA_FR)-Fwl_FR*sin(SA_FR);
Fs_RL= Fws_RL*cos(SA_RL)-Fwl_RL*sin(SA_RL);
Fs_RR= Fws_RR*cos(SA_RR)-Fwl_RR*sin(SA_RR);

%% Translation with steering Angle
Fx_FL=Fl_FL*cos(Steering_Angle)-Fs_FL*sin(Steering_Angle);
Fx_FR=Fl_FR*cos(Steering_Angle)-Fs_FR*sin(Steering_Angle);
Fx_RL=Fl_RL;
Fx_RR=Fl_RR;
y = [Fx_FL
    Fx_FR
    Fx_RL
    Fx_RR];
end

== matlab function egnition_New_updated_shiva/Tire Forces /Tire Model/Slip angle calculation/MATLAB Function ==
  data: Velocity_COG input; y output; Steering_Angle input; Yaw_Rate input; Beta input; lf input; lr input; Tf input; Tr input
function y = fcn(Velocity_COG,Steering_Angle,Yaw_Rate,Beta,lf,lr,Tf,Tr)
SA_FL= -Beta+Steering_Angle-(lf*Yaw_Rate/(Velocity_COG-0.5*Tr*Yaw_Rate));
SA_FR= -Beta+Steering_Angle-(lf*Yaw_Rate/(Velocity_COG+0.5*Tr*Yaw_Rate));
SA_RL= -Beta+(lr*Yaw_Rate/(Velocity_COG-0.5*Tr*Yaw_Rate));
SA_RR= -Beta+(lr*Yaw_Rate/(Velocity_COG+0.5*Tr*Yaw_Rate));

y = [SA_FL
    SA_FR
    SA_RL
    SA_RR];

== matlab function egnition_New_updated_shiva/Tire Forces /Tire Model/co efficient of friction calculation/MATLAB Code ==
  data: SlipL_FL input; y output; SlipL_FR input; SlipL_RL input; SlipL_RR input; SlipS_FL input; SlipS_FR input; SlipS_RL input; SlipS_RR input; SlipR_FL input; SlipR_FR input; SlipR_RL input; SlipR_RR input; FZD_FL input; FZD_FR input; FZD_RL input; FZD_RR input; Friction_Tuning_parameter input
function y = fcn(SlipL_FL,SlipL_FR,SlipL_RL,SlipL_RR,SlipS_FL,SlipS_FR,SlipS_RL,SlipS_RR,SlipR_FL,SlipR_FR,SlipR_RL,SlipR_RR,FZD_FL,FZD_FR,FZD_RL,FZD_RR,Friction_Tuning_parameter)
%added new lines
MewR_FL=Friction_Tuning_parameter*(3.0769-0.0006*FZD_FL);
MewR_FR=Friction_Tuning_parameter*(3.0769-0.0006*FZD_FR);
MewR_RL=Friction_Tuning_parameter*(3.0769-0.0006*FZD_RL);
MewR_RR=Friction_Tuning_parameter*(3.0769-0.0006*FZD_RR);
%
MewL_FL=MewR_FL*SlipL_FL/SlipR_FL;
MewL_FR=MewR_FR*SlipL_FR/SlipR_FR;
MewL_RL=MewR_RL*SlipL_RL/SlipR_RL;
MewL_RR=MewR_RR*SlipL_RR/SlipR_RR;
MewS_FL=MewR_FL*SlipS_FL/SlipR_FL;
MewS_FR=MewR_FR*SlipS_FR/SlipR_FR;
MewS_RL=MewR_RL*SlipS_RL/SlipR_RL;
MewS_RR=MewR_RR*SlipS_RR/SlipR_RR;
y=[
    MewL_FL
    MewL_FR
    MewL_RL
    MewL_RR
    MewS_FL
    MewS_FR
    MewS_RL
    MewS_RR];  

end

== matlab function egnition_New_updated_shiva/Normal Forces/Lateral Dynamic Fz/MATLAB Function1 ==
  data: l input; a_s input; W_S input; K_F input; y output; Phi input; H_s input; A_y input; Z_RF input; W_uF input; Z_uF input; K_R input; Z_RR input; W_uR input; Z_uR input; T_F input; T_R input
function y = fcn(l,a_s,W_S,K_F,Phi,H_s,A_y,Z_RF,W_uF,Z_uF,K_R,Z_RR,W_uR,Z_uR,T_F,T_R)
W_SF=((l-a_s)/l)*W_S;
W_SR=(a_s/l)*W_S;
W_F=(K_F*Phi+W_SF*H_s*Phi+W_SF*A_y*Z_RF+W_uF*A_y*Z_uF)/T_F;
W_R=(K_R*Phi+W_SR*H_s*Phi+W_SR*A_y*Z_RR+W_uR*A_y*Z_uR)/T_R;
y =[W_F
    W_R];
